simulink model "Testy"  (R2022a)
settings: Solver=VariableStepAuto  StartTime=0.0  StopTime=10.0  RelTol=1e-3
values from neighbouring files (symbols this model uses):
  A_1 = (pi * (1.2 * 15)^2) / 4 / 10000 * size^2    (= 0.101787601976)    [init.m]    (also in init_notebook.m)
  A_2 = (pi * ((1.2 * 15)^2-(1.2*5)^2)) / 4 / 10000 * size^2    (= 0.0904778684234)    [init.m]    (also in init_notebook.m)
  m = 8 * 10^(-6) * pi/4 * (5 * 1.2)^2 * 200 * size^3    (= 0.361911473694)    [init.m]    (also in init_notebook.m)
  x_max = 0.07    [init.m]    (also in init_notebook.m)
  x_min = -0.07    [init.m]    (also in init_notebook.m)
undefined symbols (not defined in the file or in its folder): p_0
settings Model: Creator=lukas  LastModifiedBy=lukas

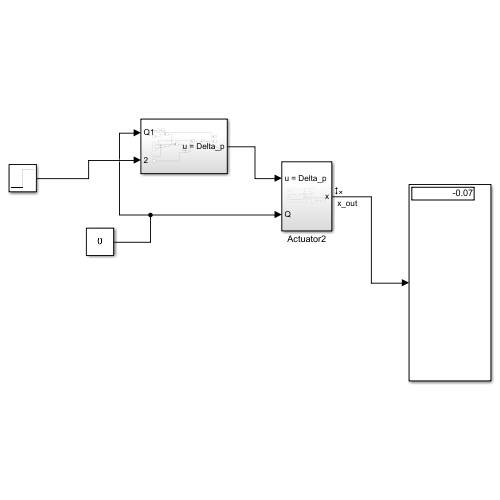
[thumbnail: Simulink's stored preview of the top-level diagram]
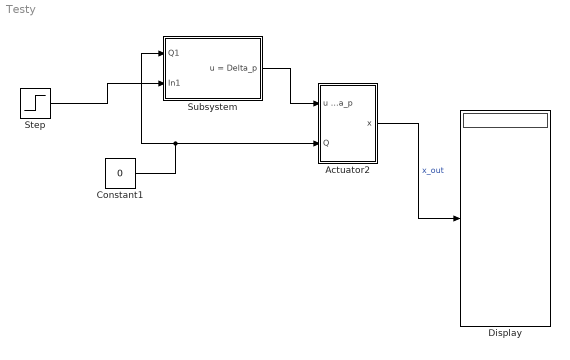
== system Testy ==
  Actuator2 : Subsystem
  Constant1 : Constant  Value=0
  Display : Display
  Step : Step  After=0.05  SampleTime=0
  Subsystem : Subsystem
  wires:
  Constant1/1 -> Subsystem/1(Q1), Actuator2/2(Q)
  Actuator2/1(x) -> Display/1  "x_out"
  Subsystem/1(u = Delta_p) -> Actuator2/1(u = Delta_p)
  Step/1 -> Subsystem/2(In1)

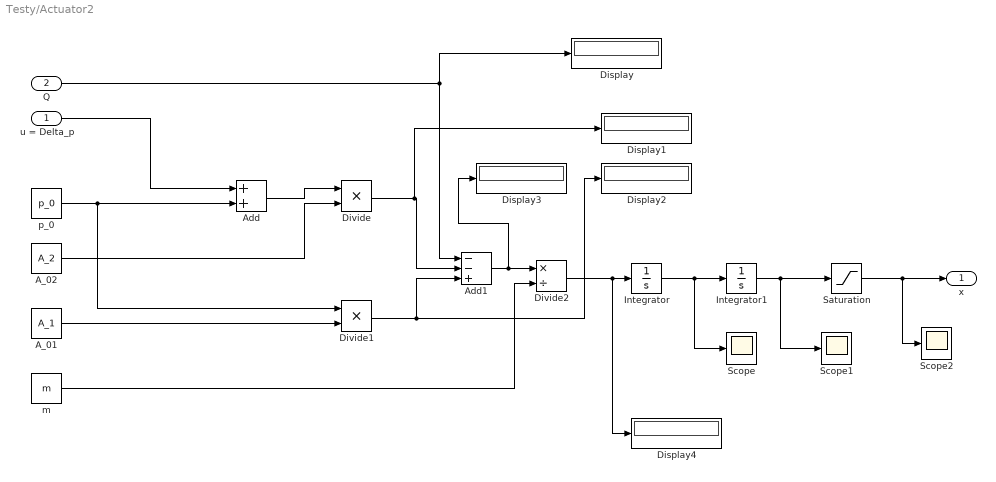
== system Testy/Actuator2 ==
  u = Delta_p : Inport
  Q : Inport  Port=2
  A_01 : Constant  Value=A_1
  A_02 : Constant  Value=A_2
  Add : Sum
  Add1 : Sum  Inputs=--+
  Display{,1..4} (5 alike) : Display
  Divide : Product  Inputs=**
  Divide1 : Product  Inputs=**
  Divide2 : Product  Inputs=*/
  Integrator : Integrator
  Integrator1 : Integrator
  Saturation : Saturate  UpperLimit=x_max  LowerLimit=x_min
  Scope : Scope
  Scope1 : Scope
  Scope2 : Scope
  m : Constant  Value=m
  p_0 : Constant  Value=p_0
  x : Outport
  wires:
  Add/1 -> Divide/1
  u = Delta_p/1 -> Add/1
  p_0/1 -> Divide1/1, Add/2
  A_02/1 -> Divide/2
  A_01/1 -> Divide1/2
  Divide/1 -> Display1/1, Add1/2
  Divide1/1 -> Display2/1, Add1/3
  Q/1 -> Add1/1, Display/1
  Add1/1 -> Display3/1, Divide2/1
  m/1 -> Divide2/2
  Divide2/1 -> Display4/1, Integrator/1
  Integrator/1 -> Scope/1, Integrator1/1
  Integrator1/1 -> Scope1/1, Saturation/1
  Saturation/1 -> Scope2/1, x/1

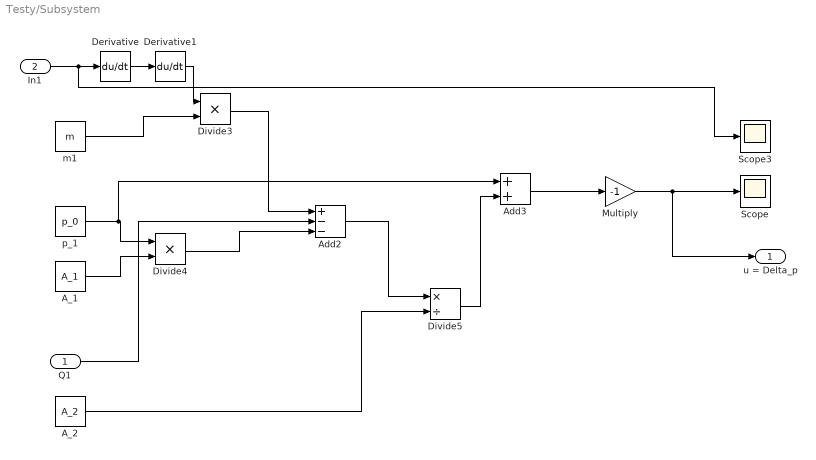
== system Testy/Subsystem ==
  Q1 : Inport
  In1 : Inport  Port=2
  A_1 : Constant  Value=A_1
  A_2 : Constant  Value=A_2
  Add2 : Sum  Inputs=+--
  Add3 : Sum
  Derivative : Derivative
  Derivative1 : Derivative
  Divide3 : Product  Inputs=**
  Divide4 : Product  Inputs=**
  Divide5 : Product  Inputs=*/
  Multiply : Gain  Gain=-1
  Scope : Scope
  Scope3 : Scope
  m1 : Constant  Value=m
  p_1 : Constant  Value=p_0
  u = Delta_p : Outport
  wires:
  Derivative1/1 -> Divide3/1
  In1/1 -> Scope3/1, Derivative/1
  m1/1 -> Divide3/2
  p_1/1 -> Add3/1, Divide4/1
  A_1/1 -> Divide4/2
  Divide3/1 -> Add2/1
  Multiply/1 -> Scope/1, u = Delta_p/1
  Add3/1 -> Multiply/1
  Derivative/1 -> Derivative1/1
  Add2/1 -> Divide5/1
  Divide4/1 -> Add2/3
  A_2/1 -> Divide5/2
  Q1/1 -> Add2/2
  Divide5/1 -> Add3/2
